simulink library "helperLibrary"  (R2020a)
settings: Solver=VariableStepAuto  StartTime=0.0  StopTime=10.0  RelTol=1e-3
values from neighbouring files (symbols this model uses):
  g = 9.8    [code.m]    (also in main.m)
  J = 2e-3    (= 0.002)    [code.m]    (also in main.m = 0.0023)
  J_R = 1e-5    (= 1e-05)    [code.m]    (also in main.m)
  m = 0.11    [code.m]    (also in main.m)
  R = 1    [code.m]    (also in main.m = 200)
  x_0 = [0.4 0.2 deg2rad(1) deg2rad(0.3)]    [code.m]    (also in main.m)
settings Model: Creator=danth  LastModifiedBy=danth

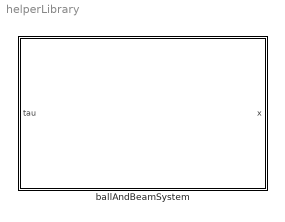
== system helperLibrary ==
  ballAndBeamSystem : Subsystem

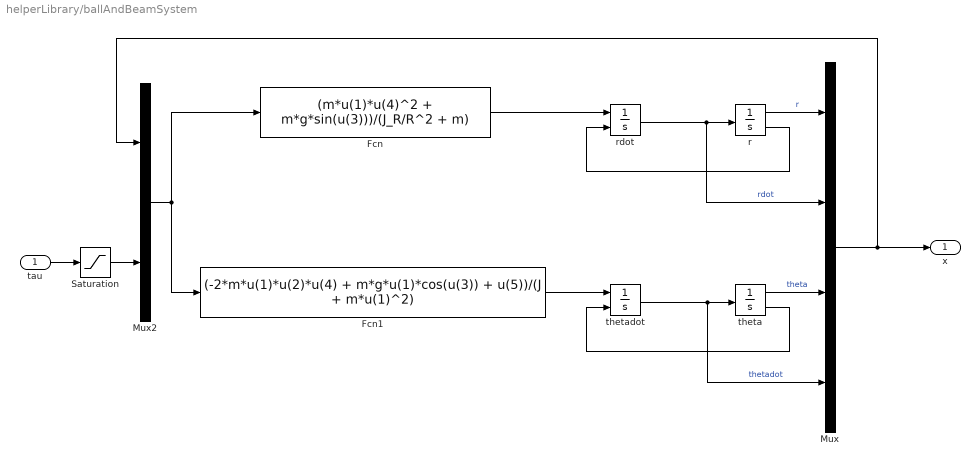
== system helperLibrary/ballAndBeamSystem ==
  tau : Inport
  Fcn : Fcn  Expr=(m*u(1)*u(4)^2 + m*g*sin(u(3)))/(J_R/R^2 + m)
  Fcn1 : Fcn  Expr=(-2*m*u(1)*u(2)*u(4) + m*g*u(1)*cos(u(3)) + u(5))/(J + m*u(1)^2)
  Mux : Mux
  Mux2 : Mux  Inputs=2
  Saturation : Saturate  UpperLimit=1  LowerLimit=-1
  r : Integrator  InitialCondition=x_0(1)  LimitOutput=on  UpperSaturationLimit=0.5  LowerSaturationLimit=-0.5  ShowSaturationPort=on
  rdot : Integrator  ExternalReset=level hold  InitialCondition=x_0(2)
  theta : Integrator  InitialCondition=x_0(3)  LimitOutput=on  UpperSaturationLimit=deg2rad(80)  LowerSaturationLimit=-deg2rad(80)  ShowSaturationPort=on
  thetadot : Integrator  ExternalReset=level hold  InitialCondition=x_0(4)
  x : Outport
  wires:
  r/1 -> Mux/1  "r"
  thetadot/1 -> theta/1, Mux/4  "thetadot"
  rdot/1 -> r/1, Mux/2  "rdot"
  tau/1 -> Saturation/1
  theta/1 -> Mux/3  "theta"
  Fcn/1 -> rdot/1
  Fcn1/1 -> thetadot/1
  Mux2/1 -> Fcn/1, Fcn1/1
  Mux/1 -> Mux2/1, x/1
  Saturation/1 -> Mux2/2
  r/2 -> rdot/2
  theta/2 -> thetadot/2
